simulink model "mrsMultiRobotSensorModel"  (R2019a)
settings: Solver=FixedStepAuto  StartTime=0.0  StopTime=30  FixedStep=sampleTime  RelTol=1e-3
PreLoadFcn:
  | % Simulation parameters
  | load exampleMap
  | sampleTime = 0.05;
  | 
  | % Lidar parameters
  | sensorOffset = [0,0];
  | scanAngles = [-3*pi/8;-pi/4;-pi/8;0;pi/8;pi/4;3*pi/8];
  | maxRange = 6;
  | 
  | % Object Detector parameters
  | objX = 4;
  | objY = 4;
  | targetLabel = 1;
  | objLabel = 1;
  | objDetectorOffset = [0 0];
  | objDetectorAngle = 0;
  | objDetectorFOV = pi/3;
  | objDetectorRange = 5;
  | objDetectorColors = [1 0 0;0 1 0;0 0 1];
  | objDetectorMaxHits = 3;
libraries: mobileRoboticsLib x9
settings Model: EnablePacing=on  Creator=scastro  LastModifiedBy=scastro
settings DataIOCC: ReturnWorkspaceOutputs=off
settings DebuggingCC: PregeneratedLibrarySubsystemCodeDiagnostic=none  ArithmeticOperatorsInVariantConditions=warning
settings SFSimCC: SimUseLocalCustomCode=off
settings RTWCC: RTWUseLocalCustomCode=off

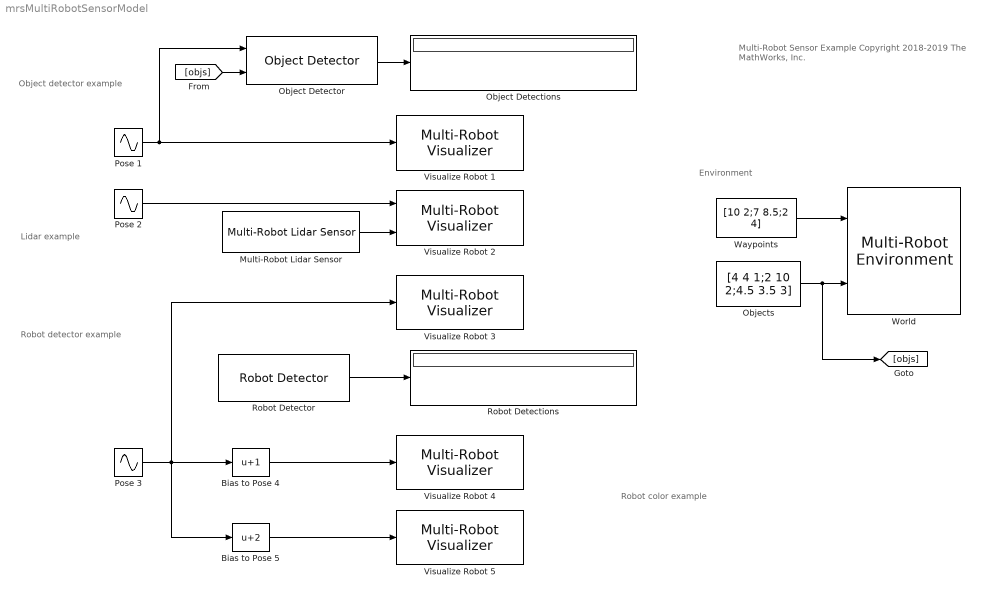
== system mrsMultiRobotSensorModel ==
  note: Robot detector example
  note: Environment
  note: Lidar example
  note: Object detector example
  note: Multi-Robot Sensor Example
      |
      | Copyright 2018-2019 The MathWorks, Inc.
  note: Robot color example
  Bias to Pose 4 : Bias  Bias=1
  Bias to Pose 5 : Bias  Bias=2
  Multi-Robot Lidar Sensor : mobileRoboticsLib/Environments/Multi-Robot Lidar Sensor  robotIdx=2  mapName=map  sensorOffset=sensorOffset  scanAngles=scanAngles  maxRange=maxRange
      settings: SourceProductName=Mobile Robotics Simulation Toolbox
  Object Detections : Display
  Object Detector : mobileRoboticsLib/Environments/Object Detector  mapName=map  sensorOffset=objDetectorOffset  sensorAngle=objDetectorAngle  fieldOfView=objDetectorFOV  maxRange=objDetectorRange  maxDetections=objDetectorMaxHits  sampleTime=-1
      settings: SourceProductName=Mobile Robotics Simulation Toolbox
  Objects : Constant  Value=[4 4 1;2 10 2;4.5 3.5 3]
  Pose 1 : Sin  SineType=Sample based  Amplitude=[1;1.5;pi/4]  Bias=[2;2;0]  Phase=[0;pi/2;0]  Samples=200  SampleTime=sampleTime
  Pose 2 : Sin  SineType=Sample based  Amplitude=[-1.5;1;2*pi/3]  Bias=[10;10;-pi/3]  Phase=[0;pi/2;0]  Samples=150  SampleTime=sampleTime
  Pose 3 : Sin  SineType=Sample based  Amplitude=[-2;0.5;pi/2]  Bias=[7.75;3;0]  Phase=[-pi/4;0;pi/3]  Samples=160  SampleTime=sampleTime  Offset=[0;50;25]
  Robot Detections : Display
  Robot Detector : mobileRoboticsLib/Environments/Robot Detector  mapName=map  robotIdx=3  sensorOffset=[ 0, 0 ]  sensorAngle=0  sensorFOV=pi/3  maxRange=10  maxDetections=3  sampleTime=-1
      settings: SourceProductName=Mobile Robotics Simulation Toolbox
  Visualize Robot 1 : mobileRoboticsLib/Environments/Multi-Robot Visualizer  idx=1  radius=0  robotColor=[0 0 1]  showTraj=off  hasLidar=off  sensorOffset=sensorOffset  scanAngles=scanAngles  maxNumScans=0  hasObjDetector=on  objDetectorOffset=objDetectorOffset  objDetectorAngle=objDetectorAngle  objDetectorFOV=objDetectorFOV  objDetectorMaxRange=objDetectorRange  hasRobotDetector=off  robotDetectorOffset=[0,0]  robotDetectorAngle=0  robotDetectorFOV=pi/3  robotDetectorMaxRange=5  robotDetectorNumDetections=0
      settings: SourceProductName=Mobile Robotics Simulation Toolbox
  Visualize Robot 2 : mobileRoboticsLib/Environments/Multi-Robot Visualizer  idx=2  radius=0.5  robotColor=[0 0 1]  showTraj=off  hasLidar=on  sensorOffset=sensorOffset  scanAngles=scanAngles  maxNumScans=0  hasObjDetector=off  objDetectorOffset=objDetectorOffset  objDetectorAngle=objDetectorAngle  objDetectorFOV=objDetectorFOV  objDetectorMaxRange=objDetectorRange  hasRobotDetector=off  robotDetectorOffset=[0,0]  robotDetectorAngle=0  robotDetectorFOV=pi/3  robotDetectorMaxRange=5  robotDetectorNumDetections=0
      settings: SourceProductName=Mobile Robotics Simulation Toolbox
  Visualize Robot 3 : mobileRoboticsLib/Environments/Multi-Robot Visualizer  idx=3  radius=0.25  robotColor=[0 0 1]  showTraj=on  hasLidar=off  sensorOffset=sensorOffset  scanAngles=scanAngles  maxNumScans=0  hasObjDetector=off  objDetectorOffset=objDetectorOffset  objDetectorAngle=objDetectorAngle  objDetectorFOV=objDetectorFOV  objDetectorMaxRange=objDetectorRange  hasRobotDetector=on  robotDetectorOffset=[0,0]  robotDetectorAngle=0  robotDetectorFOV=pi/3  robotDetectorMaxRange=10  robotDetectorNumDetections=0
      settings: SourceProductName=Mobile Robotics Simulation Toolbox
  Visualize Robot 4 : mobileRoboticsLib/Environments/Multi-Robot Visualizer  idx=4  radius=0.5  robotColor=[0 0.8 0]  showTraj=off  hasLidar=off  sensorOffset=sensorOffset  scanAngles=scanAngles  maxNumScans=0  hasObjDetector=off  objDetectorOffset=objDetectorOffset  objDetectorAngle=objDetectorAngle  objDetectorFOV=objDetectorFOV  objDetectorMaxRange=objDetectorRange  hasRobotDetector=off  robotDetectorOffset=[0,0]  robotDetectorAngle=0  robotDetectorFOV=pi/3  robotDetectorMaxRange=5  robotDetectorNumDetections=0
      settings: SourceProductName=Mobile Robotics Simulation Toolbox
  Visualize Robot 5 : mobileRoboticsLib/Environments/Multi-Robot Visualizer  idx=5  radius=0.25  robotColor=[0.6 0 0]  showTraj=off  hasLidar=off  sensorOffset=sensorOffset  scanAngles=scanAngles  maxNumScans=0  hasObjDetector=off  objDetectorOffset=objDetectorOffset  objDetectorAngle=objDetectorAngle  objDetectorFOV=objDetectorFOV  objDetectorMaxRange=objDetectorRange  hasRobotDetector=off  robotDetectorOffset=[0,0]  robotDetectorAngle=0  robotDetectorFOV=pi/3  robotDetectorMaxRange=5  robotDetectorNumDetections=0
      settings: SourceProductName=Mobile Robotics Simulation Toolbox
  Waypoints : Constant  Value=[10 2;7 8.5;2 4]
  World : mobileRoboticsLib/Environments/Multi-Robot Environment  numRobots=5  mapName=map  showWaypoints=on  showObjects=on  objectColors=[1 0 0;0 1 0;0 0 1]  objectMarkers='so^'  showRobotIds=on  plotSensorLines=on
      settings: SourceProductName=Mobile Robotics Simulation Toolbox
  wires:
  Pose 1/1 -> Object Detector/1, Visualize Robot 1/1
  Waypoints/1 -> World/1
  Objects/1 -> World/2, [objs]
  Pose 2/1 -> Visualize Robot 2/1
  Pose 3/1 -> Visualize Robot 3/1, Bias to Pose 5/1, Bias to Pose 4/1
  Multi-Robot Lidar Sensor/1 -> Visualize Robot 2/2
  [objs] -> Object Detector/2
  Object Detector/1 -> Object Detections/1
  Bias to Pose 4/1 -> Visualize Robot 4/1
  Bias to Pose 5/1 -> Visualize Robot 5/1
  Robot Detector/1 -> Robot Detections/1
